simulink model "Collision_avoidance_joystick_sensors"  (R2022b)
settings: Solver=FixedStepAuto  StartTime=0.0  StopTime=inf  RelTol=1e-3
model workspace (MAT data in the model file):
  Logfile_Data_Object = robotics.ros.BagSelection
  Logfile_Data_Object.FilePath = 'D:\Shared_Folder\test5.bag'
  Logfile_Data_Object.StartTime = 1676475449.62
  Logfile_Data_Object.EndTime = 1676475524.94
  Logfile_Data_Object.NumMessages = 5910
  Logfile_Data_Object.AvailableTopics = table
  Logfile_Data_Object.AvailableTopics.data{1} = [1; 750; 750; 455; 1; 1; 1; 751; 750; 750; 480; 469; 751]
  Logfile_Data_Object.AvailableTopics.data{2} = categorical
  Logfile_Data_Object.AvailableTopics.data{2}.categoryNames = {'dynamic_reconfigure/Config'; 'dynamic_reconfigure/ConfigDescription'; 'geometry_msgs/Twist'; 'nav_msgs/Odometry'; 'rosaria/BumperState'; 'rosgraph_msgs/Log'; 'sensor_msgs/PointCloud'; 'sensor_msgs/PointCloud2'; 'std_msgs/Bool'; 'std_msgs/Float64'; 'std_msgs/Int8'; 'tf2_msgs/TFMessage'}
  Logfile_Data_Object.AvailableTopics.data{2}.codes = [11; 10; 5; 3; 9; 2; 1; 4; 7; 8; 6; 6; 12]
  Logfile_Data_Object.AvailableTopics.data{3}{1} = 'int8 Data
    | '
  Logfile_Data_Object.AvailableTopics.data{3}{2} = 'double Data
    | '
  Logfile_Data_Object.AvailableTopics.data{3}{3} = 'std_msgs/Header Header
    |   uint32 Seq
    |   Time Stamp
    |   char FrameId
    | logical[] FrontBumpers
    | logical[] RearBumpers
    | '
  Logfile_Data_Object.AvailableTopics.data{3}{4} = 'geometry_msgs/Vector3 Linear
    |   double X
    |   double Y
    |   double Z
    | geometry_msgs/Vector3 Angular
    |   double X
    |   double Y
    |   double Z
    | '
  Logfile_Data_Object.AvailableTopics.data{3}{5} = 'logical Data
    | '
  Logfile_Data_Object.AvailableTopics.data{3}{6} = 'dynamic_reconfigure/Group[] Groups
    |   char Name
    |   char Type
    |   dynamic_reconfigure/ParamDescription[] Parameters
    |     char Name
    |     char Type
    |     uint32 Level
    |     char Description
    |     char EditMethod
    |   int32 Parent
    |   int32 Id
    | dynamic_reconfigure/Config Max
    |   dynamic_reconfigure/BoolParameter[] Bools
    |     char Name
    |     logical Value
    |   dynamic_reconfigure/IntParameter[] Ints
    |     char Name
    |     int32 Value
    |   dynamic_reconfigure/StrParameter[] Strs
    |     char Name
    |     char Value
    |   dynamic_reconfigure/DoubleParameter[] Doubles
    |     char Name
    |     double Value
    |   dynamic_reconfigure/GroupState[] Groups
    |     char Name
    |     logical State
    |     int32 Id
    |     int32 Parent
    | dynamic_reconfigure/Config Min
    |   dynamic_reconfigure/BoolParameter[] Bools
    |     char Name
    |     logical Value
    |   dynamic_reconfigure/IntParameter[] Ints
    |     char Name
    |     int32 Value
    |   dynamic_reconfigure/StrParameter[] Strs
    |     char Name
    |     char Value
    |   dynamic_reconfigure/DoubleParameter[] Doubles
    |     char Name
    |     double Value
    |   dynamic_reconfigure/GroupState[] Groups
    |     char Name
    |     logical State
    |     int32 Id
    |     int32 Parent
    | dynamic_reconfigure/Config Dflt
    |   dynamic_reconfigure/BoolParameter[] Bools
    |     char Name
    |     logical Value
    |   dynamic_reconfigure/IntParameter[] Ints
    |     char Name
    |     int32 Value
    |   dynamic_reconfigure/StrParameter[] Strs
    |     char Name
    |     char Value
    |   dynamic_reconfigure/DoubleParameter[] Doubles
    |     char Name
    |     double Value
    |   dynamic_reconfigure/GroupState[] Groups
    |     char Name
    |     logical State
    |     int32 Id
    |     int32 Parent
    | '
  Logfile_Data_Object.AvailableTopics.data{3}{7} = 'dynamic_reconfigure/BoolParameter[] Bools
    |   char Name
    |   logical Value
    | dynamic_reconfigure/IntParameter[] Ints
    |   char Name
    |   int32 Value
    | dynamic_reconfigure/StrParameter[] Strs
    |   char Name
    |   char Value
    | dynamic_reconfigure/DoubleParameter[] Doubles
    |   char Name
    |   double Value
    | dynamic_reconfigure/GroupState[] Groups
    |   char Name
    |   logical State
    |   int32 Id
    |   int32 Parent
    | '
  Logfile_Data_Object.AvailableTopics.data{3}{8} = 'std_msgs/Header Header
    |   uint32 Seq
    |   Time Stamp
    |   char FrameId
    | char ChildFrameId
    | geometry_msgs/PoseWithCovariance Pose
    |   geometry_msgs/Pose Pose
    |     geometry_msgs/Point Position
    |       double X
    |       double Y
    |       double Z
    |     geometry_msgs/Quaternion Orientation
    |       double X
    |       double Y
    |       double Z
    |       double W
    |   double[36] Covariance
    | geometry_msgs/TwistWithCovariance Twist
    |   geometry_msgs/Twist Twist
    |     geometry_msgs/Vector3 Linear
    |       double X
    |       double Y
    |       double Z
    |     geometry_msgs/Vector3 Angular
    |       double X
    |       double Y
    |       double Z
    |   double[36] Covariance
    | '
  Logfile_Data_Object.AvailableTopics.data{3}{9} = 'std_msgs/Header Header
    |   uint32 Seq
    |   Time Stamp
    |   char FrameId
    | geometry_msgs/Point32[] Points
    |   single X
    |   single Y
    |   single Z
    | sensor_msgs/ChannelFloat32[] Channels
    |   char Name
    |   single[] Values
    | '
  Logfile_Data_Object.AvailableTopics.data{3}{10} = 'std_msgs/Header Header
    |   uint32 Seq
    |   Time Stamp
    |   char FrameId
    | uint32 Height
    | uint32 Width
    | sensor_msgs/PointField[] Fields
    |   uint8 INT8
    |   uint8 UINT8
    |   uint8 INT16
    |   uint8 UINT16
    |   uint8 INT32
    |   uint8 UINT32
    |   uint8 FLOAT32
    |   uint8 FLOAT64
    |   char Name
    |   uint32 Offset
    |   uint8 Datatype
    |   uint32 Count
    | logical IsBigendian
    | uint32 PointStep
    | uint32 RowStep
    | uint8[] Data
    | logical IsDense
    | '
  Logfile_Data_Object.AvailableTopics.data{3}{11} = 'int8 DEBUG
    | int8 INFO
    | int8 WARN
    | int8 ERROR
    | int8 FATAL
    | std_msgs/Header Header
    |   uint32 Seq
    |   Time Stamp
    |   char FrameId
    | int8 Level
    | char Name
    | char Msg
    | char File
    | char Function
    | uint32 Line
    | char[] Topics
    | '
  Logfile_Data_Object.AvailableTopics.data{3}{12} = 'int8 DEBUG
    | int8 INFO
    | int8 WARN
    | int8 ERROR
    | int8 FATAL
    | std_msgs/Header Header
    |   uint32 Seq
    |   Time Stamp
    |   char FrameId
    | int8 Level
    | char Name
    | char Msg
    | char File
    | char Function
    | uint32 Line
    | char[] Topics
    | '
  Logfile_Data_Object.AvailableTopics.data{3}{13} = 'geometry_msgs/TransformStamped[] Transforms
    |   std_msgs/Header Header
    |     uint32 Seq
    |     Time Stamp
    |     char FrameId
    |   char ChildFrameId
    |   geometry_msgs/Transform Transform
    |     geometry_msgs/Vector3 Translation
    |       double X
    |       double Y
    |       double Z
    |     geometry_msgs/Quaternion Rotation
    |       double X
    |       double Y
    |       double Z
    |       double W
    | '
  Logfile_Data_Object.AvailableTopics.ndims = 2
  Logfile_Data_Object.AvailableTopics.nrows = 13
  Logfile_Data_Object.AvailableTopics.rownames = {'/RosAria/battery_recharge_state'; '/RosAria/battery_voltage'; '/RosAria/bumper_state'; '/RosAria/cmd_vel'; '/RosAria/motors_state'; '/RosAria/parameter_descriptions'; '/RosAria/parameter_updates'; '/RosAria/pose'; '/RosAria/sonar'; '/RosAria/sonar_pointcloud2'; '/rosout'; '/rosout_agg'; '/tf'}
  Logfile_Data_Object.AvailableTopics.nvars = 3
  Logfile_Data_Object.AvailableTopics.varnames = {'NumMessages', 'MessageType', 'MessageDefinition'}
  Logfile_Data_Object.AvailableTopics.props.useVariableNamesOriginal = 0
  Logfile_Data_Object.AvailableTopics.props.useDimensionNamesOriginal = 0
  Logfile_Data_Object.AvailableTopics.props.CustomProps = struct()
  Logfile_Data_Object.AvailableTopics.props.VariableCustomProps = struct()
  Logfile_Data_Object.AvailableTopics.props.versionSavedFrom = 4
  Logfile_Data_Object.AvailableTopics.props.minCompatibleVersion = 1
  Logfile_Data_Object.AvailableTopics.props.incompatibilityMsg = ''
  Logfile_Data_Object.AvailableTopics.props.VersionSavedFrom = 4
  Logfile_Data_Object.AvailableTopics.props.Description = ''
  Logfile_Data_Object.AvailableTopics.props.VariableNamesOriginal = {}
  Logfile_Data_Object.AvailableTopics.props.DimensionNames = {'Row', 'Variables'}
  Logfile_Data_Object.AvailableTopics.props.DimensionNamesOriginal = {}
  Logfile_Data_Object.AvailableTopics.props.UserData = []
  Logfile_Data_Object.AvailableTopics.props.VariableDescriptions = {}
  Logfile_Data_Object.AvailableTopics.props.VariableUnits = {}
  Logfile_Data_Object.AvailableTopics.props.VariableContinuity = {}
  Logfile_Data_Object.AvailableFrames = {'base_link'; 'odom'}
  Logfile_Data_Object.MessageList = table
  Logfile_Data_Object.MessageList.data{1} = [1676475449.62 1676475449.62 1676475449.62 1676475449.62 1676475449.62 1676475449.62 1676475449.62 1676475449.62 1676475449.62 1676475449.62 1676475449.62 1676475449.84 ... (5910 elements, 5910x1)]
  Logfile_Data_Object.MessageList.data{2} = categorical
  Logfile_Data_Object.MessageList.data{2}.categoryNames = {'/RosAria/battery_recharge_state'; '/RosAria/battery_voltage'; '/RosAria/bumper_state'; '/RosAria/cmd_vel'; '/RosAria/motors_state'; '/RosAria/parameter_descriptions'; '/RosAria/parameter_updates'; '/RosAria/pose'; '/RosAria/sonar'; '/RosAria/sonar_pointcloud2'; '/rosout'; '/rosout_agg'; '/tf'}
  Logfile_Data_Object.MessageList.data{2}.codes = [11 11 11 11 11 11 11 11 11 11 11 1 ... (5910 elements, 5910x1)]
  Logfile_Data_Object.MessageList.data{3} = categorical
  Logfile_Data_Object.MessageList.data{3}.categoryNames = {'std_msgs/Int8'; 'std_msgs/Float64'; 'rosaria/BumperState'; 'geometry_msgs/Twist'; 'std_msgs/Bool'; 'dynamic_reconfigure/ConfigDescription'; 'dynamic_reconfigure/Config'; 'nav_msgs/Odometry'; 'sensor_msgs/PointCloud'; 'sensor_msgs/PointCloud2'; 'rosgraph_msgs/Log'; 'tf2_msgs/TFMessage'}
  Logfile_Data_Object.MessageList.data{3}.codes = [11 11 11 11 11 11 11 11 11 11 11 1 ... (5910 elements, 5910x1)]
  Logfile_Data_Object.MessageList.data{4} = [5486 5741 6006 6279 6545 6823 7099 7382 7666 7939 8222 8744 ... (5910 elements, 5910x1)]
  Logfile_Data_Object.MessageList.ndims = 2
  Logfile_Data_Object.MessageList.nrows = 5910
  Logfile_Data_Object.MessageList.nvars = 4
  Logfile_Data_Object.MessageList.varnames = {'Time', 'Topic', 'MessageType', 'FileOffset'}
  Logfile_Data_Object.MessageList.props.useVariableNamesOriginal = 0
  Logfile_Data_Object.MessageList.props.useDimensionNamesOriginal = 0
  Logfile_Data_Object.MessageList.props.CustomProps = struct()
  Logfile_Data_Object.MessageList.props.VariableCustomProps = struct()
  Logfile_Data_Object.MessageList.props.versionSavedFrom = 4
  Logfile_Data_Object.MessageList.props.minCompatibleVersion = 1
  Logfile_Data_Object.MessageList.props.incompatibilityMsg = ''
  Logfile_Data_Object.MessageList.props.VersionSavedFrom = 4
  Logfile_Data_Object.MessageList.props.Description = ''
  Logfile_Data_Object.MessageList.props.VariableNamesOriginal = {}
  Logfile_Data_Object.MessageList.props.DimensionNames = {'Row', 'Variables'}
  Logfile_Data_Object.MessageList.props.DimensionNamesOriginal = {}
  Logfile_Data_Object.MessageList.props.UserData = []
  Logfile_Data_Object.MessageList.props.VariableDescriptions = {}
  Logfile_Data_Object.MessageList.props.VariableUnits = {}
  Logfile_Data_Object.MessageList.props.VariableContinuity = {}
  Logfile_Data_Object.RawMessageBuffer = containers.Map
  Logfile_Data_Object.RawMessageBuffer.serialization.keys = {}
  Logfile_Data_Object.RawMessageBuffer.serialization.values = {}
  Logfile_Data_Object.RawMessageBuffer.serialization.uniformity = 0
  Logfile_Data_Object.RawMessageBuffer.serialization.keyType = 'char'
  Logfile_Data_Object.RawMessageBuffer.serialization.valueType = 'any'
  Logfile_Data_Object.ImgMessageBuffer = containers.Map
  Logfile_Data_Object.ImgMessageBuffer.serialization.keys = {}
  Logfile_Data_Object.ImgMessageBuffer.serialization.values = {}
  Logfile_Data_Object.ImgMessageBuffer.serialization.uniformity = 0
  Logfile_Data_Object.ImgMessageBuffer.serialization.keyType = 'char'
  Logfile_Data_Object.ImgMessageBuffer.serialization.valueType = 'any'
  Logfile_Data_Object.TopicTypeMap = containers.Map
  Logfile_Data_Object.TopicTypeMap.serialization.keys = {'/RosAria/battery_recharge_state', '/RosAria/battery_voltage', '/RosAria/bumper_state', '/RosAria/cmd_vel', '/RosAria/motors_state', '/RosAria/parameter_descriptions', '/RosAria/parameter_updates', '/RosAria/pose', '/RosAria/sonar', '/RosAria/sonar_pointcloud2', '/rosout', '/rosout_agg', '/tf'}
  Logfile_Data_Object.TopicTypeMap.serialization.values = {'std_msgs/Int8', 'std_msgs/Float64', 'rosaria/BumperState', 'geometry_msgs/Twist', 'std_msgs/Bool', 'dynamic_reconfigure/ConfigDescription', 'dynamic_reconfigure/Config', 'nav_msgs/Odometry', 'sensor_msgs/PointCloud', 'sensor_msgs/PointCloud2', 'rosgraph_msgs/Log', 'rosgraph_msgs/Log', 'tf2_msgs/TFMessage'}
  Logfile_Data_Object.TopicTypeMap.serialization.uniformity = 1
  Logfile_Data_Object.TopicTypeMap.serialization.keyType = 'char'
  Logfile_Data_Object.TopicTypeMap.serialization.valueType = 'char'
  Logfile_Data_Object.TopicDefinitionMap = containers.Map
  Logfile_Data_Object.TopicDefinitionMap.serialization.keys = {'/RosAria/battery_recharge_state', '/RosAria/battery_voltage', '/RosAria/bumper_state', '/RosAria/cmd_vel', '/RosAria/motors_state', '/RosAria/parameter_descriptions', '/RosAria/parameter_updates', '/RosAria/pose', '/RosAria/sonar', '/RosAria/sonar_pointcloud2', '/rosout', '/rosout_agg', '/tf'}
  Logfile_Data_Object.TopicDefinitionMap.serialization.values{1} = 'int8 Data
    | '
  Logfile_Data_Object.TopicDefinitionMap.serialization.values{2} = 'double Data
    | '
  Logfile_Data_Object.TopicDefinitionMap.serialization.values{3} = 'std_msgs/Header Header
    |   uint32 Seq
    |   Time Stamp
    |   char FrameId
    | logical[] FrontBumpers
    | logical[] RearBumpers
    | '
  Logfile_Data_Object.TopicDefinitionMap.serialization.values{4} = 'geometry_msgs/Vector3 Linear
    |   double X
    |   double Y
    |   double Z
    | geometry_msgs/Vector3 Angular
    |   double X
    |   double Y
    |   double Z
    | '
  Logfile_Data_Object.TopicDefinitionMap.serialization.values{5} = 'logical Data
    | '
  Logfile_Data_Object.TopicDefinitionMap.serialization.values{6} = 'dynamic_reconfigure/Group[] Groups
    |   char Name
    |   char Type
    |   dynamic_reconfigure/ParamDescription[] Parameters
    |     char Name
    |     char Type
    |     uint32 Level
    |     char Description
    |     char EditMethod
    |   int32 Parent
    |   int32 Id
    | dynamic_reconfigure/Config Max
    |   dynamic_reconfigure/BoolParameter[] Bools
    |     char Name
    |     logical Value
    |   dynamic_reconfigure/IntParameter[] Ints
    |     char Name
    |     int32 Value
    |   dynamic_reconfigure/StrParameter[] Strs
    |     char Name
    |     char Value
    |   dynamic_reconfigure/DoubleParameter[] Doubles
    |     char Name
    |     double Value
    |   dynamic_reconfigure/GroupState[] Groups
    |     char Name
    |     logical State
    |     int32 Id
    |     int32 Parent
    | dynamic_reconfigure/Config Min
    |   dynamic_reconfigure/BoolParameter[] Bools
    |     char Name
    |     logical Value
    |   dynamic_reconfigure/IntParameter[] Ints
    |     char Name
    |     int32 Value
    |   dynamic_reconfigure/StrParameter[] Strs
    |     char Name
    |     char Value
    |   dynamic_reconfigure/DoubleParameter[] Doubles
    |     char Name
    |     double Value
    |   dynamic_reconfigure/GroupState[] Groups
    |     char Name
    |     logical State
    |     int32 Id
    |     int32 Parent
    | dynamic_reconfigure/Config Dflt
    |   dynamic_reconfigure/BoolParameter[] Bools
    |     char Name
    |     logical Value
    |   dynamic_reconfigure/IntParameter[] Ints
    |     char Name
    |     int32 Value
    |   dynamic_reconfigure/StrParameter[] Strs
    |     char Name
    |     char Value
    |   dynamic_reconfigure/DoubleParameter[] Doubles
    |     char Name
    |     double Value
    |   dynamic_reconfigure/GroupState[] Groups
    |     char Name
    |     logical State
    |     int32 Id
    |     int32 Parent
    | '
  Logfile_Data_Object.TopicDefinitionMap.serialization.values{7} = 'dynamic_reconfigure/BoolParameter[] Bools
    |   char Name
    |   logical Value
    | dynamic_reconfigure/IntParameter[] Ints
    |   char Name
    |   int32 Value
    | dynamic_reconfigure/StrParameter[] Strs
    |   char Name
    |   char Value
    | dynamic_reconfigure/DoubleParameter[] Doubles
    |   char Name
    |   double Value
    | dynamic_reconfigure/GroupState[] Groups
    |   char Name
    |   logical State
    |   int32 Id
    |   int32 Parent
    | '
  Logfile_Data_Object.TopicDefinitionMap.serialization.values{8} = 'std_msgs/Header Header
    |   uint32 Seq
    |   Time Stamp
    |   char FrameId
    | char ChildFrameId
    | geometry_msgs/PoseWithCovariance Pose
    |   geometry_msgs/Pose Pose
    |     geometry_msgs/Point Position
    |       double X
    |       double Y
    |       double Z
    |     geometry_msgs/Quaternion Orientation
    |       double X
    |       double Y
    |       double Z
    |       double W
    |   double[36] Covariance
    | geometry_msgs/TwistWithCovariance Twist
    |   geometry_msgs/Twist Twist
    |     geometry_msgs/Vector3 Linear
    |       double X
    |       double Y
    |       double Z
    |     geometry_msgs/Vector3 Angular
    |       double X
    |       double Y
    |       double Z
    |   double[36] Covariance
    | '
  Logfile_Data_Object.TopicDefinitionMap.serialization.values{9} = 'std_msgs/Header Header
    |   uint32 Seq
    |   Time Stamp
    |   char FrameId
    | geometry_msgs/Point32[] Points
    |   single X
    |   single Y
    |   single Z
    | sensor_msgs/ChannelFloat32[] Channels
    |   char Name
    |   single[] Values
    | '
  Logfile_Data_Object.TopicDefinitionMap.serialization.values{10} = 'std_msgs/Header Header
    |   uint32 Seq
    |   Time Stamp
    |   char FrameId
    | uint32 Height
    | uint32 Width
    | sensor_msgs/PointField[] Fields
    |   uint8 INT8
    |   uint8 UINT8
    |   uint8 INT16
    |   uint8 UINT16
    |   uint8 INT32
    |   uint8 UINT32
    |   uint8 FLOAT32
    |   uint8 FLOAT64
    |   char Name
    |   uint32 Offset
    |   uint8 Datatype
    |   uint32 Count
    | logical IsBigendian
    | uint32 PointStep
    | uint32 RowStep
    | uint8[] Data
    | logical IsDense
    | '
  Logfile_Data_Object.TopicDefinitionMap.serialization.values{11} = 'int8 DEBUG
    | int8 INFO
    | int8 WARN
    | int8 ERROR
    | int8 FATAL
    | std_msgs/Header Header
    |   uint32 Seq
    |   Time Stamp
    |   char FrameId
    | int8 Level
    | char Name
    | char Msg
    | char File
    | char Function
    | uint32 Line
    | char[] Topics
    | '
  Logfile_Data_Object.TopicDefinitionMap.serialization.values{12} = 'int8 DEBUG
    | int8 INFO
    | int8 WARN
    | int8 ERROR
    | int8 FATAL
    | std_msgs/Header Header
    |   uint32 Seq
    |   Time Stamp
    |   char FrameId
    | int8 Level
    | char Name
    | char Msg
    | char File
    | char Function
    | uint32 Line
    | char[] Topics
    | '
  Logfile_Data_Object.TopicDefinitionMap.serialization.values{13} = 'geometry_msgs/TransformStamped[] Transforms
    |   std_msgs/Header Header
    |     uint32 Seq
    |     Time Stamp
    |     char FrameId
    |   char ChildFrameId
    |   geometry_msgs/Transform Transform
    |     geometry_msgs/Vector3 Translation
    |       double X
    |       double Y
    |       double Z
    |     geometry_msgs/Quaternion Rotation
    |       double X
    |       double Y
    |       double Z
    |       double W
    | '
  Logfile_Data_Object.TopicDefinitionMap.serialization.uniformity = 1
  Logfile_Data_Object.TopicDefinitionMap.serialization.keyType = 'char'
  Logfile_Data_Object.TopicDefinitionMap.serialization.valueType = 'char'
  Logfile_Data_Object.messageTypeMap = containers.Map
  Logfile_Data_Object.messageTypeMap.serialization.keys = {}
  Logfile_Data_Object.messageTypeMap.serialization.values = {}
  Logfile_Data_Object.messageTypeMap.serialization.uniformity = 0
  Logfile_Data_Object.messageTypeMap.serialization.keyType = 'char'
  Logfile_Data_Object.messageTypeMap.serialization.valueType = 'any'
  Logfile_Data_Object.Parser = robotics.ros.internal.tf.TransformationTreeParser
  Logfile_Data_Object.Parser.UseObjectMsg = 1
  Logfile_Path = 'D:\Shared_Folder\test5.bag'
  Logfile_Playback_Duration = nan
  Logfile_Playback_Offset = nan
  SL_ROS_VariableLengthArrays_MaxSizes.CommonInfo.ArrayTruncateAction = 'EmitWarning'
  SL_ROS_VariableLengthArrays_MaxSizes.MsgTypeMap = containers.Map
  SL_ROS_VariableLengthArrays_MaxSizes.MsgTypeMap.serialization.keys = {'sensor_msgs/PointCloud2'}
  SL_ROS_VariableLengthArrays_MaxSizes.MsgTypeMap.serialization.values{1}(1).PropertyName = 'Data'
  SL_ROS_VariableLengthArrays_MaxSizes.MsgTypeMap.serialization.values{1}(1).DataType = 'uint8'
  SL_ROS_VariableLengthArrays_MaxSizes.MsgTypeMap.serialization.values{1}(1).MaxLength = 192
  SL_ROS_VariableLengthArrays_MaxSizes.MsgTypeMap.serialization.values{1}(2).PropertyName = 'Fields'
  SL_ROS_VariableLengthArrays_MaxSizes.MsgTypeMap.serialization.values{1}(2).DataType = 'sensor_msgs/PointField'
  SL_ROS_VariableLengthArrays_MaxSizes.MsgTypeMap.serialization.values{1}(2).MaxLength = 16
  SL_ROS_VariableLengthArrays_MaxSizes.MsgTypeMap.serialization.uniformity = 0
  SL_ROS_VariableLengthArrays_MaxSizes.MsgTypeMap.serialization.keyType = 'char'
  SL_ROS_VariableLengthArrays_MaxSizes.MsgTypeMap.serialization.valueType = 'any'
undefined symbols (not defined in the file): Angular, Linear
libraries: robotlib x6
settings Model: Creator=Prashanth  LastModifiedBy=Prashanth
settings OptimizationCC: EnhancedBackFolding=on  PassReuseOutputArgsAs=Individual arguments  ZeroExternalMemoryAtStartup=off  ZeroInternalMemoryAtStartup=off  MaxStackSize=64  OptimizeBlockOrder=speed  DifferentSizesBufferReuse=on  OptimizationCustomize=off  EfficientTunableParamExpr=on
settings DebuggingCC: ParameterTunabilityLossMsg=error
settings HardwareCC: ProdBitPerPointer=32  ProdBitPerSizeT=32  ProdBitPerPtrDiffT=32  ProdLargestAtomicFloat=None  ProdIntDivRoundTo=Undefined  ProdEndianess=Unspecified  ProdWordSize=32  ProdHWDeviceType=Generic->Unspecified (assume 32-bit Generic)
settings SFSimCC: MATLABDynamicMemAlloc=off
settings RTWCC: Description=Embedded Coder  SystemTargetFile=ert.tlc  HardwareBoard=Robot Operating System (ROS)  TLCOptions="-aInlineSetEventsForThisBaseRateFcn=TLC_FALSE -aSuppressMultiTaskScheduler=TLC_FALSE  -aRateBasedStepFcn=0"  TemplateMakefile=ert_default_tmf  Toolchain=Catkin  TargetLang=C++
settings CodeAppCC: ForceParamTrailComments=on  IgnoreCustomStorageClasses=off  OperatorAnnotations=on  SimulinkDataObjDesc=on  SFDataObjDesc=on  InsertBlockDesc=on

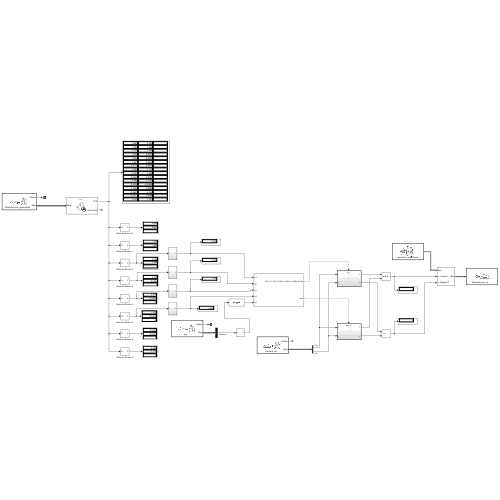
[thumbnail: Simulink's stored preview of the top-level diagram]
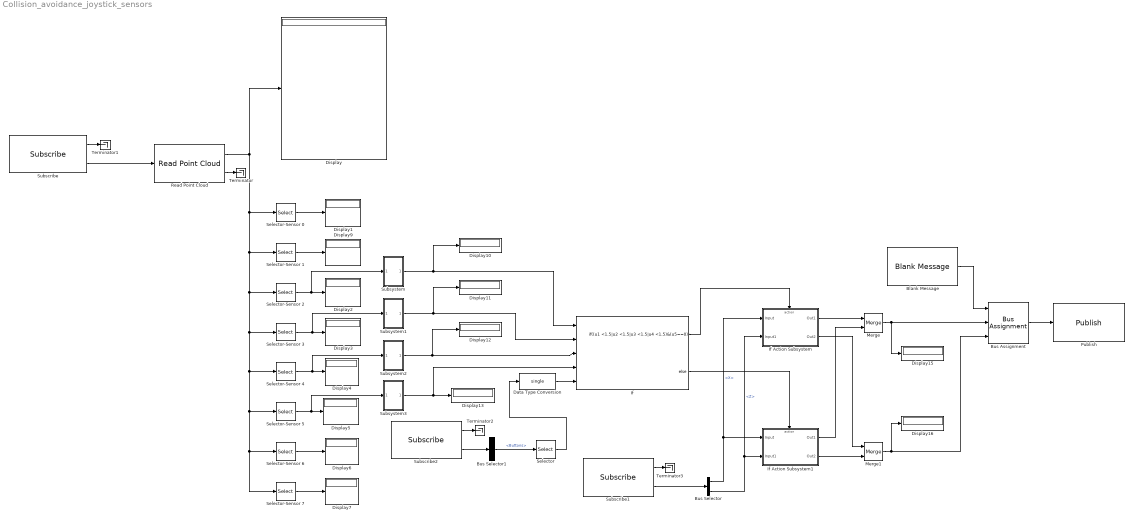
== system Collision_avoidance_joystick_sensors ==
  Blank Message : robotlib/Blank Message  messageClass=Message  entityType=geometry_msgs/Twist  messageType=geometry_msgs/Twist  SampleTime=inf  legacyBusStruct=off
      settings: LibrarySourceBlock=roslib/ROS/Blank Message
  Bus Assignment : BusAssignment  AssignedSignals=Linear.X,Angular.Z
  Bus Selector : BusSelector  OutputSignals=Linear.X,Angular.Z
  Bus Selector1 : BusSelector  OutputSignals=Buttons
  Data Type Conversion : DataTypeConversion  OutDataTypeStr=single  SaturateOnIntegerOverflow=off  RndMeth=Floor
  Display{,1..7,9..13,15..16} (15 alike) : Display
  If : If  NumInputs=5  IfExpression=(u1 <1.5|u2 <1.5|u3 <1.5|u4 <1.5)&(u5==0)
  If Action Subsystem : Subsystem  TreatAsAtomicUnit=on
  If Action Subsystem1 : Subsystem  TreatAsAtomicUnit=on
  Merge : Merge
  Merge1 : Merge
  Publish : robotlib/Publish  topicSource=Specify your own  topic=/RosAria/cmd_vel  messageType=geometry_msgs/Twist  legacyBusStruct=off  messageQueueLength=1
      settings: LibrarySourceBlock=roslib/ROS/Publish
  Read Point Cloud : robotlib/Read Point Cloud  MaximumPointCloudSize=[ 16,1 ]  PreserveStructure=off  ShowRGBOutput=off  ShowIntensityOutput=off  ShowErrorCodeOutput=on  VariableSizeOutputs=off
      settings: LibrarySourceBlock=roslib/ROS/Read Point Cloud
  Selector : Selector  NumberOfDimensions=2  InputPortWidth=3  IndexOptions=Starting index (dialog),Starting index (dialog)  Indices=1,5  OutputSizes=1,1
  Selector-Sensor 0 : Selector  NumberOfDimensions=2  IndexMode=Zero-based  InputPortWidth=8  IndexOptions=Starting index (dialog),Starting index (dialog)  Indices=0,0  OutputSizes=1,3
  Selector-Sensor 1 : Selector  NumberOfDimensions=2  IndexMode=Zero-based  InputPortWidth=6  IndexOptions=Starting index (dialog),Starting index (dialog)  Indices=1,0  OutputSizes=1,3
  Selector-Sensor 2 : Selector  NumberOfDimensions=2  IndexMode=Zero-based  InputPortWidth=6  IndexOptions=Starting index (dialog),Starting index (dialog)  Indices=2,0  OutputSizes=1,3
  Selector-Sensor 3 : Selector  NumberOfDimensions=2  IndexMode=Zero-based  InputPortWidth=6  IndexOptions=Starting index (dialog),Starting index (dialog)  Indices=3,0  OutputSizes=1,3
  Selector-Sensor 4 : Selector  NumberOfDimensions=2  IndexMode=Zero-based  InputPortWidth=6  IndexOptions=Starting index (dialog),Starting index (dialog)  Indices=4,0  OutputSizes=1,3
  Selector-Sensor 5 : Selector  NumberOfDimensions=2  IndexMode=Zero-based  InputPortWidth=6  IndexOptions=Starting index (dialog),Starting index (dialog)  Indices=5,0  OutputSizes=1,3
  Selector-Sensor 6 : Selector  NumberOfDimensions=2  IndexMode=Zero-based  InputPortWidth=7  IndexOptions=Starting index (dialog),Starting index (dialog)  Indices=6,0  OutputSizes=1,3
  Selector-Sensor 7 : Selector  NumberOfDimensions=2  IndexMode=Zero-based  InputPortWidth=7  IndexOptions=Starting index (dialog),Starting index (dialog)  Indices=7,0  OutputSizes=1,3
  Subscribe : robotlib/Subscribe  topicSource=Specify your own  topic=/RosAria/sonar_pointcloud2  messageType=sensor_msgs/PointCloud2  SampleTime=-1  legacyBusStruct=off  messageQueueLength=1
      settings: LibrarySourceBlock=roslib/ROS/Subscribe
  Subscribe1 : robotlib/Subscribe  topicSource=Specify your own  topic=/joy/cmd_vel  messageType=geometry_msgs/Twist  SampleTime=-1  legacyBusStruct=off  messageQueueLength=1
      settings: LibrarySourceBlock=roslib/ROS/Subscribe
  Subscribe2 : robotlib/Subscribe  topicSource=Specify your own  topic=/joy  messageType=sensor_msgs/Joy  SampleTime=-1  legacyBusStruct=off  messageQueueLength=1
      settings: LibrarySourceBlock=roslib/ROS/Subscribe
  Subsystem : Subsystem
  Subsystem1 : Subsystem
  Subsystem2 : Subsystem
  Subsystem3 : Subsystem
  Terminator{,1..3} (4 alike) : Terminator
  wires:
  Read Point Cloud/2 -> Terminator/1
  Read Point Cloud/1 -> Selector-Sensor 7/1, Selector-Sensor 6/1, Selector-Sensor 5/1, Selector-Sensor 4/1, Selector-Sensor 3/1, Selector-Sensor 2/1, Selector-Sensor 1/1, Selector-Sensor 0/1, Display/1
  Subscribe/2 -> Read Point Cloud/1
  Subscribe/1 -> Terminator1/1
  Selector-Sensor 0/1 -> Display1/1
  Selector-Sensor 1/1 -> Display9/1
  Selector-Sensor 2/1 -> Subsystem/1(In1), Display2/1
  Selector-Sensor 3/1 -> Subsystem1/1(In1), Display3/1
  Selector-Sensor 4/1 -> Subsystem2/1(In1), Display4/1
  Selector-Sensor 5/1 -> Subsystem3/1(In1), Display5/1
  Selector-Sensor 6/1 -> Display6/1
  Selector-Sensor 7/1 -> Display7/1
  Subsystem1/1(Out1) -> Display11/1, If/2
  Subsystem2/1(Out1) -> Display12/1, If/3
  Subsystem3/1(Out1) -> If/4, Display13/1
  If/1 -> If Action Subsystem/Action
  Bus Selector/1 -> If Action Subsystem/1(Input), If Action Subsystem1/1(Input)  "<X>"
  Bus Selector/2 -> If Action Subsystem/2(Input1), If Action Subsystem1/2(Input1)  "<Z>"
  If Action Subsystem/2(Out2) -> Merge1/1
  Subsystem/1(Out1) -> If/1, Display10/1
  If Action Subsystem/1(Out1) -> Merge/1
  If Action Subsystem1/1(Out1) -> Merge/2
  If Action Subsystem1/2(Out2) -> Merge1/2
  Merge1/1 -> Display16/1, Bus Assignment/3
  Bus Assignment/1 -> Publish/1
  Merge/1 -> Display15/1, Bus Assignment/2
  Blank Message/1 -> Bus Assignment/1
  Subscribe1/2 -> Bus Selector/1
  Subscribe2/2 -> Bus Selector1/1
  Bus Selector1/1 -> Selector/1  "<Buttons>"
  Selector/1 -> Data Type Conversion/1
  Subscribe2/1 -> Terminator2/1
  Subscribe1/1 -> Terminator3/1
  Data Type Conversion/1 -> If/5
  If/2 -> If Action Subsystem1/Action

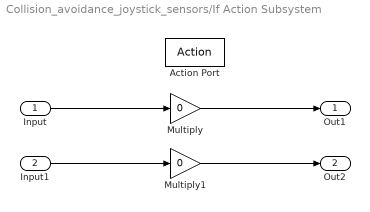
== system Collision_avoidance_joystick_sensors/If Action Subsystem ==
  Input : Inport
  Input1 : Inport  Port=2
  Action Port : ActionPort  ActionPortLabel=if((u1 <2|u2 <2|u3 <2|u4 <2)&(u5==0))
  Multiply : Gain  Gain=0
  Multiply1 : Gain  Gain=0
  Out1 : Outport
  Out2 : Outport  Port=2
  wires:
  Multiply1/1 -> Out2/1
  Input1/1 -> Multiply1/1
  Input/1 -> Multiply/1
  Multiply/1 -> Out1/1

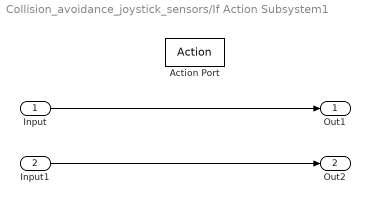
== system Collision_avoidance_joystick_sensors/If Action Subsystem1 ==
  Input : Inport
  Input1 : Inport  Port=2
  Action Port : ActionPort  ActionPortLabel=else
  Out1 : Outport
  Out2 : Outport  Port=2
  wires:
  Input1/1 -> Out2/1
  Input/1 -> Out1/1

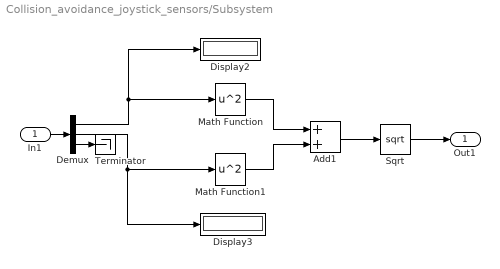
== system Collision_avoidance_joystick_sensors/Subsystem ==
  In1 : Inport
  Add1 : Sum
  Demux : Demux  Outputs=3
  Display2 : Display
  Display3 : Display
  Math Function : Math  Operator=square
  Math Function1 : Math  Operator=square
  Sqrt : Sqrt
  Terminator : Terminator
  Out1 : Outport
  wires:
  Math Function1/1 -> Add1/2
  Demux/1 -> Math Function/1, Display2/1
  In1/1 -> Demux/1
  Math Function/1 -> Add1/1
  Demux/2 -> Display3/1, Math Function1/1
  Sqrt/1 -> Out1/1
  Add1/1 -> Sqrt/1
  Demux/3 -> Terminator/1

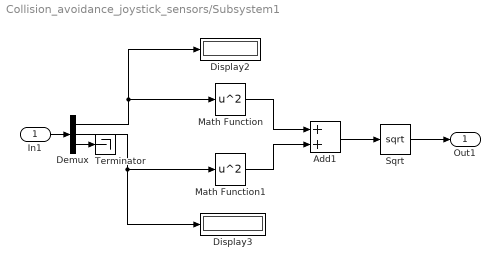
== system Collision_avoidance_joystick_sensors/Subsystem1 ==
  In1 : Inport
  Add1 : Sum
  Demux : Demux  Outputs=3
  Display2 : Display
  Display3 : Display
  Math Function : Math  Operator=square
  Math Function1 : Math  Operator=square
  Sqrt : Sqrt
  Terminator : Terminator
  Out1 : Outport
  wires:
  Math Function1/1 -> Add1/2
  Demux/1 -> Math Function/1, Display2/1
  In1/1 -> Demux/1
  Math Function/1 -> Add1/1
  Demux/2 -> Display3/1, Math Function1/1
  Sqrt/1 -> Out1/1
  Add1/1 -> Sqrt/1
  Demux/3 -> Terminator/1

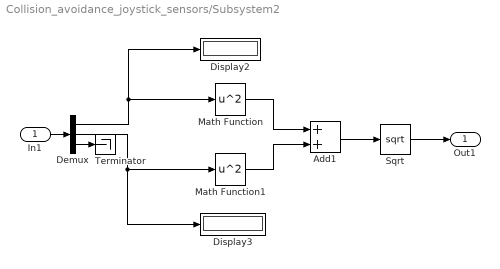
== system Collision_avoidance_joystick_sensors/Subsystem2 ==
  In1 : Inport
  Add1 : Sum
  Demux : Demux  Outputs=3
  Display2 : Display
  Display3 : Display
  Math Function : Math  Operator=square
  Math Function1 : Math  Operator=square
  Sqrt : Sqrt
  Terminator : Terminator
  Out1 : Outport
  wires:
  Math Function1/1 -> Add1/2
  Demux/1 -> Math Function/1, Display2/1
  In1/1 -> Demux/1
  Math Function/1 -> Add1/1
  Demux/2 -> Display3/1, Math Function1/1
  Sqrt/1 -> Out1/1
  Add1/1 -> Sqrt/1
  Demux/3 -> Terminator/1

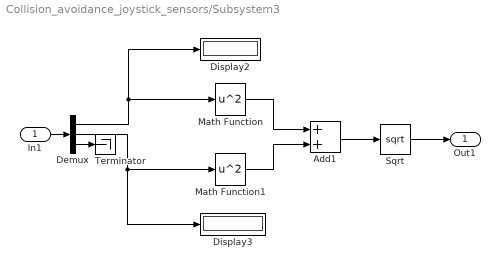
== system Collision_avoidance_joystick_sensors/Subsystem3 ==
  In1 : Inport
  Add1 : Sum
  Demux : Demux  Outputs=3
  Display2 : Display
  Display3 : Display
  Math Function : Math  Operator=square
  Math Function1 : Math  Operator=square
  Sqrt : Sqrt
  Terminator : Terminator
  Out1 : Outport
  wires:
  Math Function1/1 -> Add1/2
  Demux/1 -> Math Function/1, Display2/1
  In1/1 -> Demux/1
  Math Function/1 -> Add1/1
  Demux/2 -> Display3/1, Math Function1/1
  Sqrt/1 -> Out1/1
  Add1/1 -> Sqrt/1
  Demux/3 -> Terminator/1
